simulink model "sampleModel2043"  (R2023a)
settings: Solver=VariableStepAuto  StartTime=0.0  StopTime=10.0  RelTol=1e-3
libraries: simulink x6, hdlsllib x5
settings Model: Creator=user1  LastModifiedBy=user1

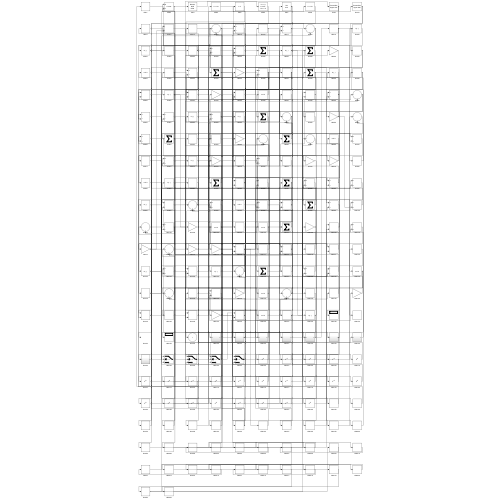
[thumbnail: Simulink's stored preview of the top-level diagram]
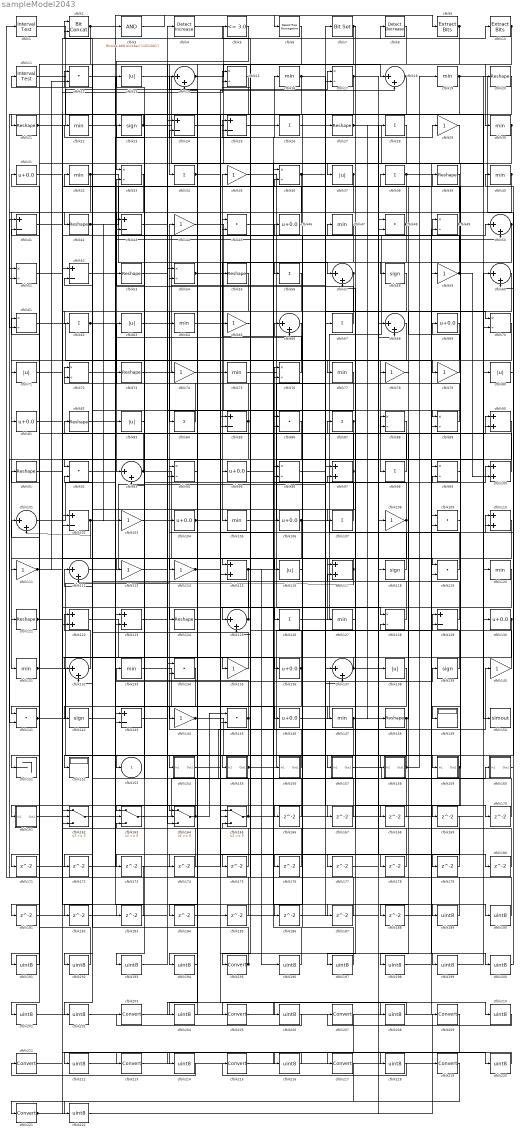
== system sampleModel2043 ==
  cfblk1 : hdlsllib/Logic and Bit Operations/Interval Test  IntervalClosedRight=on  uplimit=0.5  IntervalClosedLeft=on  lowlimit=-0.5  OutDataTypeStr=boolean
  cfblk10 : simulink/Logic and Bit Operations/Extract Bits  bitsToExtract=Upper half  numBits=8  bitIdxRange=[0 7]  outScalingMode=Preserve fixed-point scaling
      settings: LibrarySourceBlock=|
      | hdlsllib/Logic and Bit
      | Operations/Extract Bits
  cfblk{90,97,100,110,115,117,122..123} (8 alike) : Sum
  cfblk{14,18,50,57,60,66,68,93,101,112,125,132,137} (13 alike) : Sum  Inputs=|++
  cfblk{24..25,41,43,52,85,102,129,143} (9 alike) : Sum  Inputs=+-
  cfblk{29,35,44,59,65,74,78..79,103,108,111,113..114,135,140,144} (16 alike) : Gain
  cfblk{31,46,69,81,95,104,106,130,136,146} (10 alike) : Bias  Bias=0.0  SaturateOnIntegerOverflow=off
  cfblk{16,19,22,30,32,40,47,64,75,77,105,120,127,131,133,147} (16 alike) : MinMax
  cfblk{26,28,34,38,56,62,67,84,87,98,107,126} (12 alike) : Sum  Inputs=+
  cfblk{12,45,48,86,92,109,119,134,141,145} (10 alike) : DotProduct  OutDataTypeStr=Inherit: Inherit via internal rule
  cfblk11 : hdlsllib/Logic and Bit Operations/Interval Test  IntervalClosedRight=on  uplimit=0.5  IntervalClosedLeft=on  lowlimit=-0.5  OutDataTypeStr=boolean
  cfblk{13,37,63,71,80,83,116,138} (8 alike) : Abs  SaturateOnIntegerOverflow=off
  cfblk{23,58,118,139,142} (5 alike) : Signum
  cfblk{20..21,27,39,42,53,55,73,82,91,121,124,148} (13 alike) : Reshape
  cfblk{15,17,33,36,49,51,54,61,70,72,76,88..89,94,96,99,128} (17 alike) : Product  Inputs=*/  RndMeth=Zero  SaturateOnIntegerOverflow=on
  cfblk149 : Display
  cfblk150 : ToWorkspace  VariableName=simout  SaveFormat=Timeseries  SampleTime=-1
  cfblk151 : Terminator
  cfblk152 : Display
  cfblk154 : Subsystem
      settings: LibrarySourceBlock=|
      | hdlsllib/Ports &
      | Subsystems/Subsystem
  cfblk155 : Subsystem
      settings: LibrarySourceBlock=|
      | hdlsllib/Ports &
      | Subsystems/Subsystem
  cfblk156 : Subsystem
      settings: LibrarySourceBlock=|
      | hdlsllib/Ports &
      | Subsystems/Subsystem
  cfblk157 : Subsystem
      settings: LibrarySourceBlock=|
      | hdlsllib/Ports &
      | Subsystems/Subsystem
  cfblk158 : Subsystem
      settings: LibrarySourceBlock=|
      | hdlsllib/Ports &
      | Subsystems/Subsystem
  cfblk159 : Subsystem
      settings: LibrarySourceBlock=|
      | hdlsllib/Ports &
      | Subsystems/Subsystem
  cfblk160 : Subsystem
      settings: LibrarySourceBlock=|
      | hdlsllib/Ports &
      | Subsystems/Subsystem
  cfblk161 : Subsystem
      settings: LibrarySourceBlock=|
      | hdlsllib/Ports &
      | Subsystems/Subsystem
  cfblk{162..165} (4 alike) : Switch  SaturateOnIntegerOverflow=off  InputSameDT=off
  cfblk{166..188} (23 alike) : Delay  SampleTime=1
  cfblk{189..194,196..202,204,206,208,210,212,214,216,218,220,222} (23 alike) : DataTypeConversion  OutDataTypeStr=uint8  SaturateOnIntegerOverflow=off  RndMeth=Floor
  cfblk{195,203,205,207,209,211,213,215,217,219,221} (11 alike) : DataTypeConversion  SaturateOnIntegerOverflow=off  RndMeth=Floor
  cfblk2 : hdlsllib/Logic and Bit Operations/Bit Concat  numInputs=2
  cfblk3 : simulink/Logic and Bit Operations/Bitwise Operator  logicop=AND  UseBitMask=on  BitMask=bin2dec('11011001')  BitMaskRealWorld=Stored Integer
      settings: LibrarySourceBlock=|
      | hdlsllib/Logic and Bit
      | Operations/Bitwise
      | Operator
  cfblk4 : simulink/Logic and Bit Operations/Detect Increase  vinit=0.0  OutDataTypeStr=boolean
      settings: LibrarySourceBlock=|
      | hdlsllib/Logic and Bit
      | Operations/Detect
      | Increase
  cfblk5 : hdlsllib/Logic and Bit Operations/Compare To Constant  relop=<=  const=3.0  OutDataTypeStr=boolean
  cfblk6 : hdlsllib/Logic and Bit Operations/Detect Rise Nonnegative  vinit=0  OutDataTypeStr=boolean
  cfblk7 : simulink/Logic and Bit Operations/Bit Set  iBit=0
      settings: LibrarySourceBlock=|
      | hdlsllib/Logic and Bit
      | Operations/Bit Set
  cfblk8 : simulink/Logic and Bit Operations/Detect Decrease  vinit=0.0  OutDataTypeStr=boolean
      settings: LibrarySourceBlock=|
      | hdlsllib/Logic and Bit
      | Operations/Detect
      | Decrease
  cfblk9 : simulink/Logic and Bit Operations/Extract Bits  bitsToExtract=Upper half  numBits=8  bitIdxRange=[0 7]  outScalingMode=Preserve fixed-point scaling
      settings: LibrarySourceBlock=|
      | hdlsllib/Logic and Bit
      | Operations/Extract Bits
  cfblk153 : Outport  VectorParamsAs1DForOutWhenUnconnected=off
  wires:
  cfblk164/1 -> cfblk145/1, cfblk43/2, cfblk161/1(In1)
  cfblk7/1 -> cfblk34/1, cfblk37/1
  cfblk145/1 -> cfblk133/1, cfblk153/1
  cfblk32/1 -> cfblk57/1, cfblk71/1
  cfblk5/1 -> cfblk33/1
  cfblk67/1 -> cfblk33/2
  cfblk126/1 -> cfblk50/1
  cfblk19/1 -> cfblk155/1(In1), cfblk102/2, cfblk43/1
  cfblk21/1 -> cfblk17/1, cfblk15/2
  cfblk139/1 -> cfblk82/1
  cfblk123/1 -> cfblk4/1
  cfblk76/1 -> cfblk35/1
  cfblk63/1 -> cfblk49/1
  cfblk35/1 -> cfblk128/1
  cfblk165/1 -> cfblk140/1, cfblk120/1
  cfblk136/1 -> cfblk72/1, cfblk194/1
  cfblk38/1 -> cfblk93/1, cfblk107/1, cfblk200/1
  cfblk156/1(Out1) -> cfblk76/1
  cfblk59/1 -> cfblk13/1, cfblk100/2
  cfblk47/1 -> cfblk105/1
  cfblk112/1 -> cfblk17/2
  cfblk158/1(Out1) -> cfblk44/1, cfblk19/1
  cfblk69/1 -> cfblk98/1
  cfblk92/1 -> cfblk123/1
  cfblk120/1 -> cfblk163/1
  cfblk130/1 -> cfblk182/1, cfblk202/1
  cfblk68/1 -> cfblk131/1
  cfblk105/1 -> cfblk27/1
  cfblk157/1(Out1) -> cfblk160/1(In1)
  cfblk4/1 -> cfblk118/1
  cfblk30/1 -> cfblk89/1, cfblk76/2
  cfblk155/1(Out1) -> cfblk129/1, cfblk45/2
  cfblk58/1 -> cfblk83/1
  cfblk85/1 -> cfblk52/2, cfblk141/2
  cfblk61/1 -> cfblk78/1
  cfblk24/1 -> cfblk67/1
  cfblk141/1 -> cfblk54/2, cfblk91/1
  cfblk147/1 -> cfblk152/1, cfblk99/2
  cfblk122/1 -> cfblk165/1
  cfblk97/1 -> cfblk25/1, cfblk132/2
  cfblk40/1 -> cfblk144/1, cfblk125/2
  cfblk159/1(Out1) -> cfblk39/1, cfblk197/1
  cfblk140/1 -> cfblk88/1
  cfblk44/1 -> cfblk99/1
  cfblk110/1 -> cfblk121/1
  cfblk131/1 -> cfblk158/1(In1), cfblk10/1
  cfblk77/1 -> cfblk92/1
  cfblk36/1 -> cfblk164/2, cfblk164/3, cfblk170/1, cfblk204/1
  cfblk116/1 -> cfblk66/1
  cfblk143/1 -> cfblk38/1
  cfblk161/1(Out1) -> cfblk90/1
  cfblk20/1 -> cfblk135/1
  cfblk2/1 -> cfblk111/1, cfblk9/1
  cfblk3/1 -> cfblk6/1
  cfblk104/1 -> cfblk116/1, cfblk18/2
  cfblk80/1 -> cfblk40/1
  cfblk84/1 -> cfblk63/1
  cfblk99/1 -> cfblk149/1
  cfblk12/1 -> cfblk146/1
  cfblk98/1 -> cfblk72/2
  cfblk135/1 -> cfblk22/1
  cfblk107/1 -> cfblk46/1
  cfblk132/1 -> cfblk122/1
  cfblk57/1 -> cfblk115/1, cfblk96/2
  cfblk117/1 -> cfblk114/1, cfblk112/2
  cfblk129/1 -> cfblk2/1
  cfblk52/1 -> cfblk143/2
  cfblk91/1 -> cfblk122/2
  cfblk54/1 -> cfblk137/1, cfblk119/1
  cfblk11/1 -> cfblk150/1
  cfblk114/1 -> cfblk178/1, cfblk179/1
  cfblk64/1 -> cfblk79/1
  cfblk33/1 -> cfblk81/1
  cfblk62/1 -> cfblk66/2, cfblk172/1
  cfblk108/1 -> cfblk23/1, cfblk147/1
  cfblk51/1 -> cfblk95/1
  cfblk79/1 -> cfblk32/1
  cfblk9/1 -> cfblk125/1, cfblk94/2
  cfblk73/1 -> cfblk7/1
  cfblk101/1 -> cfblk50/2
  cfblk93/1 -> cfblk127/1, cfblk61/1
  cfblk148/1 -> cfblk128/2, cfblk183/1
  cfblk29/1 -> cfblk56/1
  cfblk119/1 -> cfblk94/1
  cfblk27/1 -> cfblk59/1, cfblk148/1
  cfblk50/1 -> cfblk77/1, cfblk169/1
  cfblk115/1 -> cfblk162/2, cfblk100/1, cfblk90/2, cfblk196/1
  cfblk43/1 -> cfblk8/1
  cfblk160/1(Out1) -> cfblk110/1
  cfblk154/1(Out1) -> cfblk106/1
  cfblk26/1 -> cfblk70/1
  cfblk133/1 -> cfblk156/1(In1)
  cfblk146/1 -> cfblk108/1
  cfblk10/1 -> cfblk30/1, cfblk164/1
  cfblk53/1 -> cfblk89/2
  cfblk103/1 -> cfblk138/1
  cfblk37/1 -> cfblk142/1, cfblk61/2, cfblk65/1
  cfblk13/1 -> cfblk75/1
  cfblk56/1 -> cfblk84/1
  cfblk1/1 -> cfblk85/2
  cfblk48/1 -> cfblk42/1, cfblk58/1
  cfblk45/1 -> cfblk29/1
  cfblk125/1 -> cfblk53/1, cfblk11/1
  cfblk106/1 -> cfblk110/2, cfblk145/2
  cfblk23/1 -> cfblk80/1, cfblk21/1
  cfblk83/1 -> cfblk113/1
  cfblk31/1 -> cfblk136/1
  cfblk144/1 -> cfblk159/1(In1), cfblk14/2, cfblk199/1
  cfblk94/1 -> cfblk154/1(In1)
  cfblk86/1 -> cfblk195/1
  cfblk89/1 -> cfblk45/1
  cfblk71/1 -> cfblk117/1
  cfblk87/1 -> cfblk123/2, cfblk115/2
  cfblk100/1 -> cfblk88/2
  cfblk163/1 -> cfblk68/1
  cfblk137/1 -> cfblk132/1, cfblk129/2, cfblk57/2
  cfblk22/1 -> cfblk3/1
  cfblk121/1 -> cfblk87/1, cfblk47/1
  cfblk127/1 -> cfblk97/2
  cfblk142/1 -> cfblk139/1
  cfblk18/1 -> cfblk176/1, cfblk177/1
  cfblk15/1 -> cfblk73/1
  cfblk6/1 -> cfblk62/1
  cfblk49/1 -> cfblk15/1, cfblk186/1
  cfblk14/1 -> cfblk18/1, cfblk124/1, cfblk184/1
  cfblk113/1 -> cfblk64/1
  cfblk118/1 -> cfblk96/1
  cfblk102/1 -> cfblk157/1(In1), cfblk101/2, cfblk181/1
  cfblk111/1 -> cfblk31/1, cfblk151/1, cfblk36/2, cfblk12/2
  cfblk16/1 -> cfblk141/1, cfblk70/2
  cfblk42/1 -> cfblk20/1, cfblk103/1
  cfblk65/1 -> cfblk5/1
  cfblk46/1 -> cfblk12/1
  cfblk25/1 -> cfblk16/1
  cfblk75/1 -> cfblk130/1
  cfblk34/1 -> cfblk126/1, cfblk119/2
  cfblk128/1 -> cfblk14/1
  cfblk81/1 -> cfblk102/1
  cfblk39/1 -> cfblk55/1
  cfblk162/1 -> cfblk26/1
  cfblk109/1 -> cfblk69/1
  cfblk55/1 -> cfblk162/3
  cfblk17/1 -> cfblk51/2, cfblk180/1
  cfblk88/1 -> cfblk166/1
  cfblk166/1 -> cfblk93/2
  cfblk72/1 -> cfblk167/1
  cfblk167/1 -> cfblk2/2
  cfblk96/1 -> cfblk168/1
  cfblk168/1 -> cfblk97/1
  cfblk170/1 -> cfblk143/1
  cfblk70/1 -> cfblk171/1
  cfblk171/1 -> cfblk85/1
  cfblk172/1 -> cfblk163/2
  cfblk66/1 -> cfblk173/1
  cfblk173/1 -> cfblk1/1
  cfblk138/1 -> cfblk174/1
  cfblk174/1 -> cfblk163/3
  cfblk90/1 -> cfblk175/1
  cfblk175/1 -> cfblk52/1
  cfblk176/1 -> cfblk36/1
  cfblk177/1 -> cfblk48/1
  cfblk178/1 -> cfblk165/2
  cfblk179/1 -> cfblk25/2
  cfblk180/1 -> cfblk117/2
  cfblk181/1 -> cfblk24/1
  cfblk182/1 -> cfblk54/1
  cfblk183/1 -> cfblk51/1
  cfblk184/1 -> cfblk137/2
  cfblk124/1 -> cfblk185/1
  cfblk185/1 -> cfblk112/1
  cfblk186/1 -> cfblk68/2
  cfblk82/1 -> cfblk187/1
  cfblk187/1 -> cfblk165/3
  cfblk78/1 -> cfblk188/1
  cfblk188/1 -> cfblk49/2
  cfblk41/1 -> cfblk189/1
  cfblk189/1 -> cfblk24/2
  cfblk95/1 -> cfblk190/1
  cfblk190/1 -> cfblk41/1
  cfblk8/1 -> cfblk191/1
  cfblk191/1 -> cfblk41/2
  cfblk134/1 -> cfblk192/1
  cfblk192/1 -> cfblk101/1
  cfblk169/1 -> cfblk193/1
  cfblk193/1 -> cfblk134/1
  cfblk194/1 -> cfblk134/2
  cfblk195/1 -> cfblk92/2, cfblk104/1
  cfblk196/1 -> cfblk86/1
  cfblk197/1 -> cfblk86/2
  cfblk60/1 -> cfblk198/1
  cfblk198/1 -> cfblk109/1
  cfblk199/1 -> cfblk60/1
  cfblk200/1 -> cfblk60/2
  cfblk28/1 -> cfblk201/1
  cfblk201/1 -> cfblk109/2
  cfblk202/1 -> cfblk28/1
  cfblk204/1 -> cfblk74/1
  cfblk74/1 -> cfblk206/1
  cfblk206/1 -> cfblk203/1
  cfblk203/1 -> cfblk208/1
  cfblk208/1 -> cfblk205/1
  cfblk205/1 -> cfblk210/1
  cfblk210/1 -> cfblk207/1
  cfblk207/1 -> cfblk212/1
  cfblk212/1 -> cfblk209/1
  cfblk209/1 -> cfblk214/1
  cfblk214/1 -> cfblk211/1
  cfblk211/1 -> cfblk216/1
  cfblk216/1 -> cfblk213/1
  cfblk213/1 -> cfblk218/1
  cfblk218/1 -> cfblk215/1
  cfblk219/1 -> cfblk221/1
  cfblk215/1 -> cfblk220/1
  cfblk220/1 -> cfblk217/1
  cfblk221/1 -> cfblk162/1, cfblk48/2
  cfblk217/1 -> cfblk222/1
  cfblk222/1 -> cfblk219/1

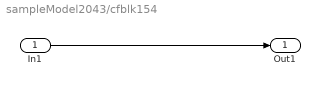
== system sampleModel2043/cfblk154 ==
  In1 : Inport
  Out1 : Outport
  wires:
  In1/1 -> Out1/1

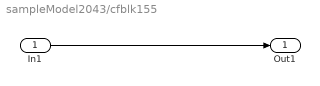
== system sampleModel2043/cfblk155 ==
  In1 : Inport
  Out1 : Outport
  wires:
  In1/1 -> Out1/1

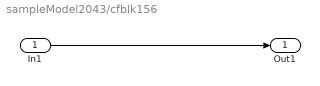
== system sampleModel2043/cfblk156 ==
  In1 : Inport
  Out1 : Outport
  wires:
  In1/1 -> Out1/1

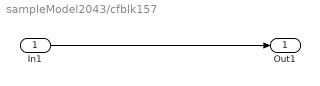
== system sampleModel2043/cfblk157 ==
  In1 : Inport
  Out1 : Outport
  wires:
  In1/1 -> Out1/1

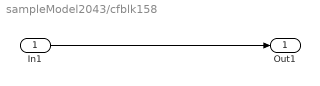
== system sampleModel2043/cfblk158 ==
  In1 : Inport
  Out1 : Outport
  wires:
  In1/1 -> Out1/1

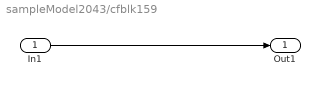
== system sampleModel2043/cfblk159 ==
  In1 : Inport
  Out1 : Outport
  wires:
  In1/1 -> Out1/1

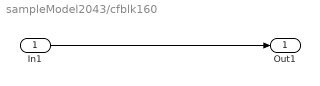
== system sampleModel2043/cfblk160 ==
  In1 : Inport
  Out1 : Outport
  wires:
  In1/1 -> Out1/1

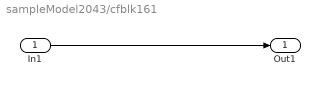
== system sampleModel2043/cfblk161 ==
  In1 : Inport
  Out1 : Outport
  wires:
  In1/1 -> Out1/1
